simulink model "untitled"  (R2022b)
settings: Solver=VariableStepAuto  StartTime=0.0  StopTime=10.0  RelTol=1e-3
libraries: simulink_extras x1
settings Model: Creator=AMD  LastModifiedBy=AMD

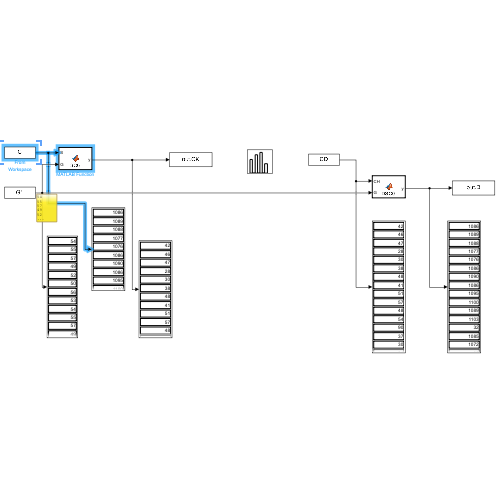
[thumbnail: Simulink's stored preview of the top-level diagram]
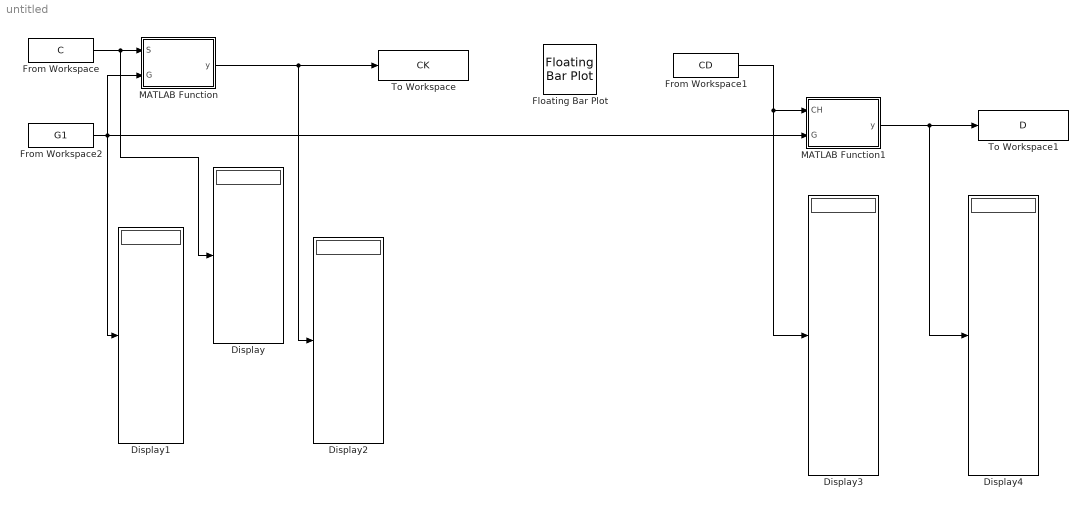
== system untitled ==
  Display{,1..4} (5 alike) : Display
  Floating Bar Plot : simulink_extras/Additional Sinks/Floating Bar Plot  yLim=[1040 1104]
  From Workspace : FromWorkspace  VariableName=C
  From Workspace1 : FromWorkspace  VariableName=CD
  From Workspace2 : FromWorkspace  VariableName=G1
  MATLAB Function : MATLAB Function  TreatAsAtomicUnit=on
  MATLAB Function1 : MATLAB Function  TreatAsAtomicUnit=on
  To Workspace : ToWorkspace  VariableName=CK  SaveFormat=Timeseries  SampleTime=-1
  To Workspace1 : ToWorkspace  VariableName=D  SaveFormat=Timeseries  SampleTime=-1
  wires:
  From Workspace/1 -> Display/1, MATLAB Function/1(S)
  From Workspace2/1 -> MATLAB Function/2(G), MATLAB Function1/2(G), Display1/1
  MATLAB Function/1(y) -> To Workspace/1, Display2/1
  MATLAB Function1/1(y) -> Display4/1, To Workspace1/1
  From Workspace1/1 -> Display3/1, MATLAB Function1/1(CH)

== matlab function untitled/MATLAB Function ==
  data: S input; y output; G input
function y = SCG(S, G)
C = double(S);
G1 = double(G);
CK = mod(C + 6 + G1, 1104);
y = CK;
y;

== matlab function untitled/MATLAB Function1 ==
  data: CH input; y output; G input
function y = DSCG(CH, G)
CD = double(CH);
G1 = double(G);
D = mod(CD - G1 - 6 + 1104, 1104);
y = D;
y;
